simulink model "FULL_1_DOF_fuzzy"  (R2024b)
settings: Solver=FixedStepAuto  StartTime=0.0  StopTime=300  FixedStep=0.002  RelTol=1e-6
undefined symbols (not defined in the file): beta, d2, D_position, I_omega, P_omega, P_position, tau_set
libraries: slpidlib x2, fuzblock x1, simulink x1
settings Model: Creator=franc  LastModifiedBy=donadi
settings OptimizationCC: BlockReduction=off  DefaultParameterBehavior=Inlined  BufferReuse=off
settings RTWCC: GPUComputeCapability=3.5

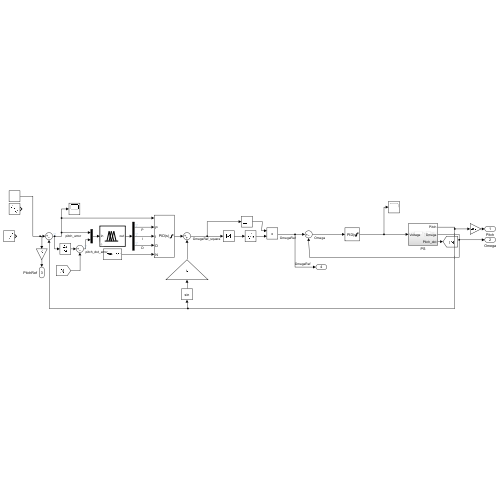
[thumbnail: Simulink's stored preview of the top-level diagram]
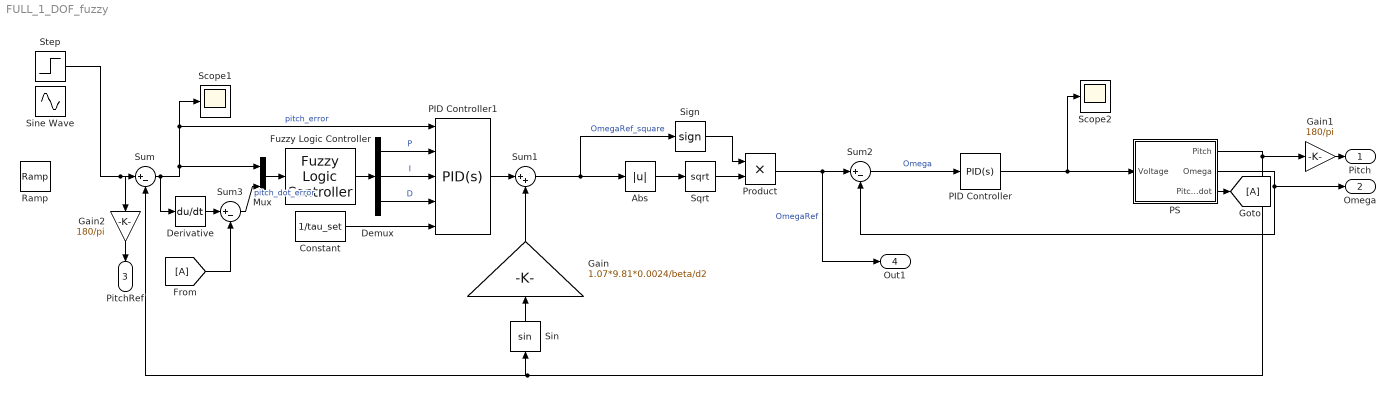
== system FULL_1_DOF_fuzzy ==
  Abs : Abs  SaturateOnIntegerOverflow=off
  Constant : Constant  Value=1/tau_set
  Demux : Demux  Outputs=3
  Derivative : Derivative
  From : From
  Fuzzy Logic Controller : fuzblock/Fuzzy Logic  Controller  FIS=sugenotype2  OutputSampleNumber=101  DataType=double  FuzzifiedInputs=off  RuleFiringStrengths=off  RuleOutputs=off  AggregatedOutputs=off  SimulateUsing=Interpreted execution  OutOfRangeInputValueMessage=warning  NoRuleFiredMessage=warning  EmptyOutputFuzzySetMessage=warning
  Gain : Gain  Gain=1.07*9.81*0.0024/beta/d2
  Gain1 : Gain  Gain=180/pi
  Gain2 : Gain  Gain=180/pi
  Goto : Goto
  Mux : Mux  Inputs=2
  PID Controller : slpidlib/PID Controller  Controller=PID  Form=Parallel  TimeDomain=Continuous-time  UseExternalTs=off  SampleTime=-1  IntegratorMethod=Forward Euler  FilterMethod=Forward Euler  ControllerParametersSource=internal  P=P_omega  I=I_omega  UseKiTs=off  D=0  UseExternalDerivativeSource=off  N=100  UseFilter=on  TunerSelectOption=Transfer Function Based (PID Tuner App)  InitialConditionSource=internal  InitialConditionForIntegrator=0  InitialConditionForFilter=0  DifferentiatorICPrevScaledInput=0  ExternalReset=none  TrackingMode=off  Kt=1  LimitOutput=on  SatLimitsSource=internal  UpperSaturationLimit=18  LowerSaturationLimit=-18  LinearizeAsGain=on  AntiWindupMode=none  Kb=1  LimitIntegrator=off  UpperIntegratorSaturationLimit=inf  LowerIntegratorSaturationLimit=-inf  POutMin=[]  POutMax=[]  IOutMin=[]  IOutMax=[]  DOutMin=[]  DOutMax=[]  NOutMin=[]  NOutMax=[]  SumOutMin=[]  SumOutMax=[]  SaturationOutMin=[]  SaturationOutMax=[]  PParamMin=[]  PParamMax=[]  IParamMin=[]  IParamMax=[]  DParamMin=[]  DParamMax=[]  NParamMin=[]  NParamMax=[]  KbParamMin=[]  KbParamMax=[]  KtParamMin=[]  KtParamMax=[]  KbOutMin=[]  KbOutMax=[]  KtOutMin=[]  KtOutMax=[]  IntegratorOutMin=[]  IntegratorOutMax=[]  FilterOutMin=[]  FilterOutMax=[]  SumI1OutMin=[]  SumI1OutMax=[]  SumI2OutMin=[]  SumI2OutMax=[]  SumI3OutMin=[]  SumI3OutMax=[]  SumI4OutMin=[]  SumI4OutMax=[]  SumDOutMin=[]  SumDOutMax=[]  DifferentiatorOutMin=[]  DifferentiatorOutMax=[]  FilterDiffOutCoefMin=[]  FilterDiffOutCoefMax=[]  ReciprocalOutMin=[]  ReciprocalOutMax=[]  SumDenOutMin=[]  SumDenOutMax=[]  SumNumOutMin=[]  SumNumOutMax=[]  DivideOutMin=[]  DivideOutMax=[]  UdiffTsProdOutMin=[]  UdiffTsProdOutMax=[]  NTsProdOutMin=[]  NTsProdOutMax=[]  UintegralTsProdOutMin=[]  UintegralTsProdOutMax=[]  UngainTsProdOutMin=[]  UngainTsProdOutMax=[]  ClampingZeroOutDataTypeStr=Inherit: Inherit via back propagation  ClampingZeroOutMin=[]  ClampingZeroOutMax=[]  FilterDenConstantOutDataTypeStr=Inherit: Inherit via back propagation  FilterDenConstantOutMin=[]  FilterDenConstantOutMax=[]  PCopyOutDataTypeStr=Inherit: Inherit via back propagation  PCopyOutMin=[]  PCopyOutMax=[]  NCopyOutDataTypeStr=Inherit: Inherit via back propagation  NCopyOutMin=[]  NCopyOutMax=[]  IntegratorContinuousStateAttributes=''  IntegratorStateMustResolveToSignalObject=off  IntegratorRTWStateStorageClass=Auto  FilterContinuousStateAttributes=''  FilterStateMustResolveToSignalObject=off  FilterRTWStateStorageClass=Auto  ParallelPVariant=InternalParameters  IdealPVariant=Disabled  IVariant=InternalParameters  DVariant=InternalParameters  IntegratorVariant=Continuous  SatVariant=Enabled  AWVariant=Passthrough  PCopyVariant=Disabled  TRVariant=Disabled  FdbkBlocksVariant=Forward  IdealPFdbkVariant=Disabled  SatFdbkVariant=Disabled  DerivativeFilterVariant=ContFilter  NVariant=InternalParameters  NCopyVariant=Disabled  FilterICVariant=InternalICsFilter  IntegratorICVariant=InternalICs  ExternalResetVariant=Disabled  TRSumVariant=Passthrough  SumFdbkVariant=Disabled  SumVariant=Sum_PID  TsampFilterVariant=InternalTs  TsampNgainVariant=Passthrough  TsampIntegralVariant=Disabled_SignalSpec  ExternalSaturationOutDataTypeStr=Inherit: Same as second input  DerivativeSourceVariant=ErrorSignal  PreIntVariant=InternalPreInt
  PID Controller1 : slpidlib/PID Controller  Controller=PID  Form=Parallel  TimeDomain=Continuous-time  UseExternalTs=off  SampleTime=1/500  IntegratorMethod=Forward Euler  FilterMethod=Forward Euler  ControllerParametersSource=external  P=P_position*40  I=5000  UseKiTs=off  D=D_position*5  UseExternalDerivativeSource=off  N=1/tau_set  UseFilter=on  TunerSelectOption=Frequency Response Based  InitialConditionSource=internal  InitialConditionForIntegrator=0  InitialConditionForFilter=0  DifferentiatorICPrevScaledInput=0  ExternalReset=none  TrackingMode=off  Kt=1  LimitOutput=on  SatLimitsSource=internal  UpperSaturationLimit=217^2  LowerSaturationLimit=-217^2  LinearizeAsGain=on  AntiWindupMode=clamping  Kb=1  LimitIntegrator=off  UpperIntegratorSaturationLimit=inf  LowerIntegratorSaturationLimit=-inf  POutMin=[]  POutMax=[]  IOutMin=[]  IOutMax=[]  DOutMin=[]  DOutMax=[]  NOutMin=[]  NOutMax=[]  SumOutMin=[]  SumOutMax=[]  SaturationOutMin=[]  SaturationOutMax=[]  PParamMin=[]  PParamMax=[]  IParamMin=[]  IParamMax=[]  DParamMin=[]  DParamMax=[]  NParamMin=[]  NParamMax=[]  KbParamMin=[]  KbParamMax=[]  KtParamMin=[]  KtParamMax=[]  KbOutMin=[]  KbOutMax=[]  KtOutMin=[]  KtOutMax=[]  IntegratorOutMin=[]  IntegratorOutMax=[]  FilterOutMin=[]  FilterOutMax=[]  SumI1OutMin=[]  SumI1OutMax=[]  SumI2OutMin=[]  SumI2OutMax=[]  SumI3OutMin=[]  SumI3OutMax=[]  SumI4OutMin=[]  SumI4OutMax=[]  SumDOutMin=[]  SumDOutMax=[]  DifferentiatorOutMin=[]  DifferentiatorOutMax=[]  FilterDiffOutCoefMin=[]  FilterDiffOutCoefMax=[]  ReciprocalOutMin=[]  ReciprocalOutMax=[]  SumDenOutMin=[]  SumDenOutMax=[]  SumNumOutMin=[]  SumNumOutMax=[]  DivideOutMin=[]  DivideOutMax=[]  UdiffTsProdOutMin=[]  UdiffTsProdOutMax=[]  NTsProdOutMin=[]  NTsProdOutMax=[]  UintegralTsProdOutMin=[]  UintegralTsProdOutMax=[]  UngainTsProdOutMin=[]  UngainTsProdOutMax=[]  ClampingZeroOutDataTypeStr=Inherit: Inherit via back propagation  ClampingZeroOutMin=[]  ClampingZeroOutMax=[]  FilterDenConstantOutDataTypeStr=Inherit: Inherit via back propagation  FilterDenConstantOutMin=[]  FilterDenConstantOutMax=[]  PCopyOutDataTypeStr=Inherit: Inherit via back propagation  PCopyOutMin=[]  PCopyOutMax=[]  NCopyOutDataTypeStr=Inherit: Inherit via back propagation  NCopyOutMin=[]  NCopyOutMax=[]  IntegratorContinuousStateAttributes=''  IntegratorStateMustResolveToSignalObject=off  IntegratorRTWStateStorageClass=Auto  FilterContinuousStateAttributes=''  FilterStateMustResolveToSignalObject=off  FilterRTWStateStorageClass=Auto  ParallelPVariant=ExternalParameters  IdealPVariant=Disabled  IVariant=ExternalParameters  DVariant=ExternalParameters  IntegratorVariant=Continuous  SatVariant=Enabled  AWVariant=ContClampingParallel  PCopyVariant=Disabled  TRVariant=Disabled  FdbkBlocksVariant=Forward  IdealPFdbkVariant=Disabled  SatFdbkVariant=Disabled  DerivativeFilterVariant=ContFilter  NVariant=ExternalParameters  NCopyVariant=Disabled  FilterICVariant=InternalICsFilter  IntegratorICVariant=InternalICs  ExternalResetVariant=Disabled  TRSumVariant=Passthrough  SumFdbkVariant=Disabled  SumVariant=Sum_PID  TsampFilterVariant=InternalTs  TsampNgainVariant=Passthrough  TsampIntegralVariant=Disabled_SignalSpec  ExternalSaturationOutDataTypeStr=Inherit: Same as second input  DerivativeSourceVariant=ErrorSignal  PreIntVariant=InternalPreInt
  PS : Subsystem
  Product : Product
  Ramp : simulink/Sources/Ramp  slope=1  start=0  InitialOutput=0
  Scope1 : Scope
  Scope2 : Scope
  Sign : Signum
  Sin : Trigonometry
  Sine Wave : Sin  Frequency=2*pi/12  SampleTime=0
  Sqrt : Sqrt
  Step : Step  After=30*pi/180  SampleTime=0
  Sum : Sum  Inputs=|+-
  Sum1 : Sum  Inputs=|++
  Sum2 : Sum  Inputs=|+-
  Sum3 : Sum  Inputs=|+-
  Pitch : Outport
  Omega : Outport  Port=2
  PitchRef : Outport  Port=3
  Out1 : Outport  Port=4
  wires:
  PS/1(Pitch) -> Sum/2, Sin/1, Gain1/1
  PS/2(Omega) -> Sum2/2, Omega/1
  Sum2/1 -> PID Controller/1  "Omega"
  Sin/1 -> Gain/1
  Sqrt/1 -> Product/2
  Abs/1 -> Sqrt/1
  Sign/1 -> Product/1
  Gain/1 -> Sum1/2
  Sum1/1 -> Abs/1, Sign/1  "OmegaRef_square"
  PID Controller/1 -> Scope2/1, PS/1(Voltage)
  Gain1/1 -> Pitch/1
  Gain2/1 -> PitchRef/1
  PID Controller1/1 -> Sum1/1
  Product/1 -> Sum2/1, Out1/1  "OmegaRef"
  Fuzzy Logic Controller/1 -> Demux/1
  Demux/1 -> PID Controller1/2  "P"
  Demux/2 -> PID Controller1/3  "I"
  Demux/3 -> PID Controller1/4  "D"
  Constant/1 -> PID Controller1/5
  PS/3(Pitch_dot) -> Goto/1
  Mux/1 -> Fuzzy Logic Controller/1
  Step/1 -> Gain2/1, Sum/1
  Sum/1 -> Derivative/1, Mux/1, PID Controller1/1, Scope1/1  "pitch_error"
  Derivative/1 -> Sum3/1
  From/1 -> Sum3/2
  Sum3/1 -> Mux/2  "pitch_dot_error"

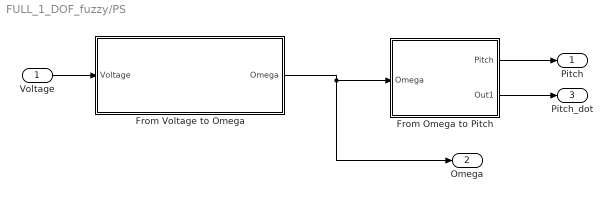
== system FULL_1_DOF_fuzzy/PS ==
  Voltage : Inport
  From Omega to Pitch : Subsystem
  From Voltage to Omega : Subsystem
  Pitch : Outport
  Omega : Outport  Port=2
  Pitch_dot : Outport  Port=3
  wires:
  From Omega to Pitch/1(Pitch) -> Pitch/1
  From Voltage to Omega/1(Omega) -> From Omega to Pitch/1(Omega), Omega/1
  Voltage/1 -> From Voltage to Omega/1(Voltage)
  From Omega to Pitch/2(Out1) -> Pitch_dot/1

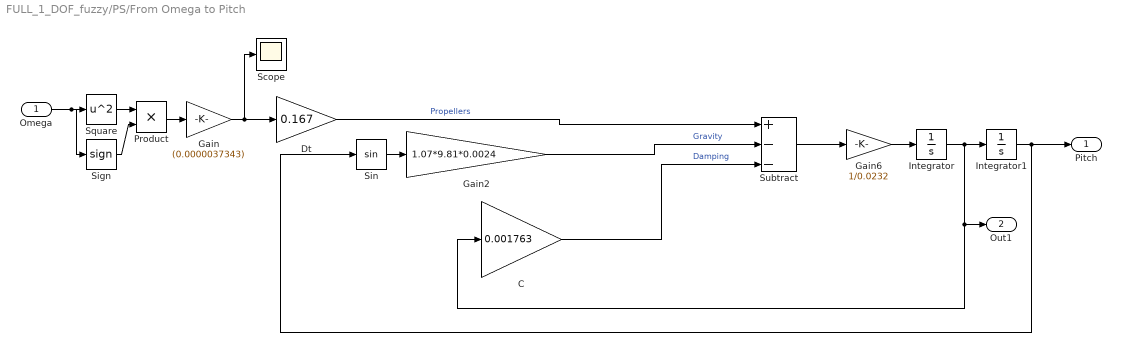
== system FULL_1_DOF_fuzzy/PS/From Omega to Pitch ==
  Omega : Inport
  C : Gain  Gain=0.001763
  Dt : Gain  Gain=0.167
  Gain : Gain  Gain=(0.0000037343)
  Gain2 : Gain  Gain=1.07*9.81*0.0024
  Gain6 : Gain  Gain=1/0.0232
  Integrator : Integrator
  Integrator1 : Integrator
  Product : Product
  Scope : Scope
  Sign : Signum  ZeroCross=off
  Sin : Trigonometry
  Square : Math  Operator=square
  Subtract : Sum  Inputs=+--
  Pitch : Outport
  Out1 : Outport  Port=2
  wires:
  Integrator1/1 -> Pitch/1, Sin/1
  Sin/1 -> Gain2/1
  Subtract/1 -> Gain6/1
  Gain2/1 -> Subtract/2  "Gravity"
  C/1 -> Subtract/3  "Damping"
  Omega/1 -> Sign/1, Square/1
  Gain6/1 -> Integrator/1
  Integrator/1 -> Integrator1/1, Out1/1, C/1
  Dt/1 -> Subtract/1  "Propellers"
  Product/1 -> Gain/1
  Square/1 -> Product/1
  Sign/1 -> Product/2
  Gain/1 -> Scope/1, Dt/1

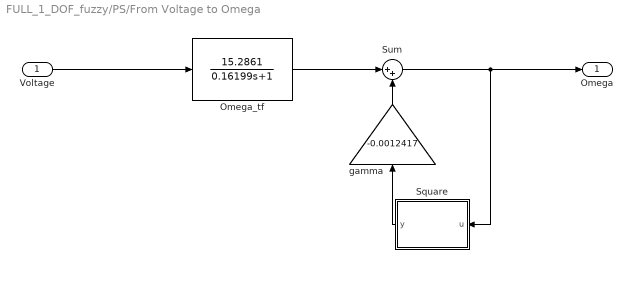
== system FULL_1_DOF_fuzzy/PS/From Voltage to Omega ==
  Voltage : Inport
  Omega_tf : TransferFcn  Numerator=15.2861  Denominator=[0.16199 1]
  Square : MATLAB Function  TreatAsAtomicUnit=on
  Sum : Sum  Inputs=|++
  gamma : Gain  Gain=-0.0012417
  Omega : Outport
  wires:
  Voltage/1 -> Omega_tf/1
  gamma/1 -> Sum/2
  Square/1(y) -> gamma/1
  Omega_tf/1 -> Sum/1
  Sum/1 -> Omega/1, Square/1(u)

== matlab function FULL_1_DOF_fuzzy/PS/From Voltage to Omega/Square ==
  data: u input; y output
function y = fcn(u)
y=u^2*sign(u);
